simulink model "MatrixAdder"  (R2017b)
settings: Solver=VariableStepAuto  StartTime=0.0  StopTime=10.0  RelTol=1e-3
settings Model: Creator=Kalana  LastModifiedBy=Kalana

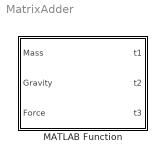
== system MatrixAdder ==
  MATLAB Function : MATLAB Function  TreatAsAtomicUnit=on

== matlab function MatrixAdder/MATLAB Function ==
  data: Mass input; t1 output; Gravity input; Force input; t2 output; t3 output
function [t1, t2, t3] = MatrixAdder(Mass, Gravity, Force)

t = Mass + Gravity;

t1 = t(1);
t2 = t(2);
t3 = t(3);
